simulink model "myexp8_3"  (R2022a)
settings: Solver=VariableStepAuto  StartTime=0.0  StopTime=10  RelTol=1e-3
undefined symbols (not defined in the file or in its folder): m, Q
libraries: commblkcod2 x2, commfilt2 x2, commdigbbndam3 x2, commchan3 x1, commrandsrc3 x1, commsink2 x1, dspsigops x1
settings Model: Creator=惠普  LastModifiedBy=惠普

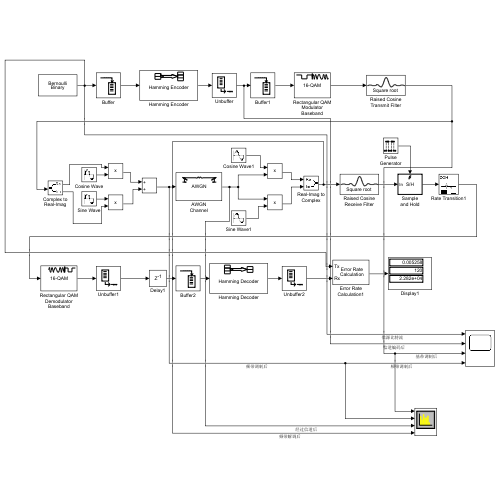
[thumbnail: Simulink's stored preview of the top-level diagram]
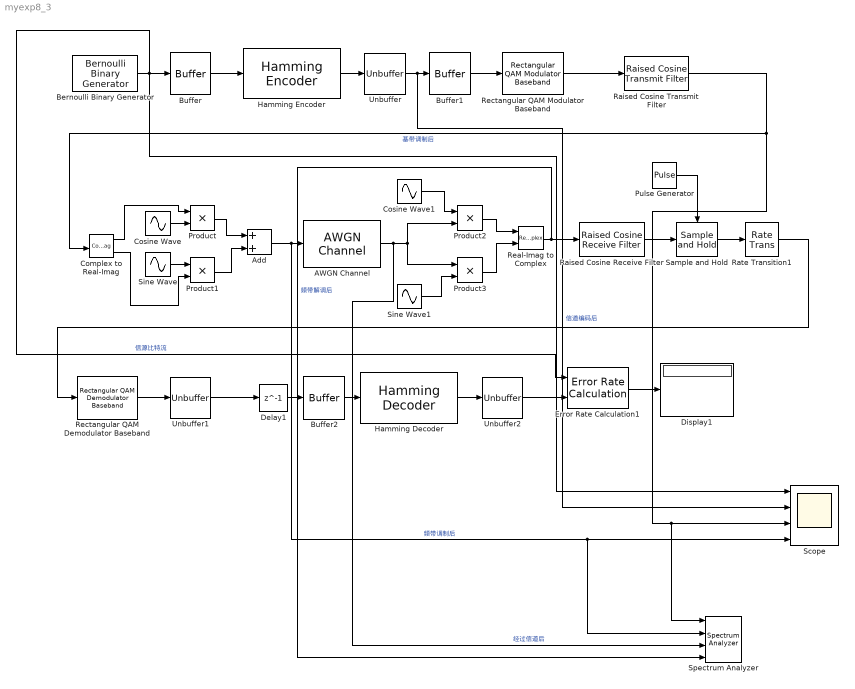
== system myexp8_3 ==
  AWGN Channel : commchan3/AWGN Channel  InputProcessing=Columns as channels (frame based)  seed=137  noiseMode="Signal to noise ratio  (Es/No)"  EbNodB=SNR  EsNodB=12  SNRdB=10  bitsPerSym=k  Ps=1  Tsym=1e-3  variance=1
  Add : Sum
  Bernoulli Binary Generator : commrandsrc3/Bernoulli Binary Generator  ProbabilityOfZero=0.5  SeedSource=Auto  Seed=0  SampleTime=1e-3*(2^m-1)/log2(Q)/(2^m-m-1)  SamplesPerFrame=1  OutputDataType=double  SimulateUsing=Interpreted execution
  Buffer : Buffer  N=2^m-m-1  OutputFrames=off
  Buffer1 : Buffer  N=log2(Q)  OutputFrames=off
  Buffer2 : Buffer  N=2^m-1  OutputFrames=off
  Complex to Real-Imag : ComplexToRealImag
  Cosine Wave : Sin  Amplitude=sqrt(2)  Frequency=2*pi*(10e3)  Phase=pi/2  SampleTime=1e-6
  Cosine Wave1 : Sin  Amplitude=sqrt(2)  Frequency=2*pi*(10e3)  Phase=pi/2  SampleTime=1e-6
  Delay1 : Delay  DelayLength=1  InitialCondition=0
  Display1 : Display
  Error Rate Calculation1 : commsink2/Error Rate Calculation  N=36  st_delay=0  cp_mode=Entire frame  subframe=[]  PMode=Port  WsName=ErrorVec  RsMode2=off  stop=off  numErr=100  maxBits=1e6
  Hamming Decoder : commblkcod2/Hamming Decoder  n=2^m-1  k=2^m-m-1
      settings: SourceProductBaseCode=CM
  Hamming Encoder : commblkcod2/Hamming Encoder  n=2^m-1  k=2^m-m-1
      settings: SourceProductBaseCode=CM
  Product{,1..3} (4 alike) : Product
  Pulse Generator : DiscretePulseGenerator  Period=1e3  PhaseDelay=10  SampleTime=1e-6
  Raised Cosine Receive Filter : commfilt2/Raised Cosine Receive Filter  filtType=Square root  R=0.5  filtSpan=10  N=1000  downFactor=1  downOffset=0  filterGain=1/sqrt(1000)  InputProcessing=Columns as channels (frame based)  RateOptions=Allow multirate processing  framing=Mute  checkCoeff=off  variableName=rcRxFilt1  currentFiltSpan=10  D=5  inputOffset=0  sampMode=Mute  saveAsFlag=0  rateMode=Downsampling  checkGain=Normalized  launchFVT=on  roundingMode=Floor  overflowMode=off  coeffDataTypeStr=Inherit: Same word length as input  coeffMin=[]  coeffMax=[]  coeffLastDataTypeStr=Inherit: Same word length as input  accumDataTypeStr=Inherit: Same as product output  accumLastDataTypeStr=Inherit: Same as product output  outputDataTypeStr=Inherit: Same as accumulator  outputMin=[]  outputMax=[]  outputLastDataTypeStr=Inherit: Same as accumulator
  Raised Cosine Transmit Filter : commfilt2/Raised Cosine Transmit Filter  filtType=Square root  R=0.5  filtSpan=10  N=1000  filterGain=sqrt(1000)  InputProcessing=Columns as channels (frame based)  RateOptions=Allow multirate processing  framing=Mute  checkCoeff=off  variableName=rcTxFilt1  checkGain=Normalized  sampMode=Mute  saveAsFlag=0  currentFiltSpan=10  D=(10)/2  launchFVT=on  roundingMode=Floor  overflowMode=off  coeffDataTypeStr=Inherit: Same word length as input  coeffMin=[]  coeffMax=[]  coeffLastDataTypeStr=Inherit: Same word length as input  outputDataTypeStr=Inherit: Same as accumulator  outputMin=[]  outputMax=[]  outputLastDataTypeStr=Inherit: Same as accumulator
  Rate Transition1 : RateTransition  OutPortSampleTime=1e-3
  Real-Imag to Complex : RealImagToComplex
  Rectangular QAM Demodulator Baseband : commdigbbndam3/Rectangular QAM Demodulator Baseband  M=Q  OutType=Bit  DecType=Hard decision  VarSource=Dialog  Variance=1  Dec=Gray  Mapping=[0:15]  PowType=Average Power  MinDist=2  AvgPow=1  PeakPow=1  Ph=0  outDtype1=Inherit via internal rule  outDtype2=Inherit via internal rule  derotateFactorWordLen=16  derotateFactorDataTypeStr=Inherit: Same word length as input  derotateFactorLastDataTypeStr=Inherit: Same word length as input  denormFactorWordLen=16  denormFactorDataTypeStr=Inherit: Same word length as input  denormFactorLastDataTypeStr=Inherit: Same word length as input  prodOutWordLen=32  prodOutOverflowMode=Wrap  prodOutRoundingMode=Floor  prodOutOvFlMode=off  prodOutOvFlModeLastStrValue=off  sumWordLen=32
  Rectangular QAM Modulator Baseband : commdigbbndam3/Rectangular QAM Modulator Baseband  M=Q  InType=Bit  Enc=Gray  Mapping=[0:15]  PowType=Average Power  MinDist=2  AvgPow=1  PeakPow=1  Ph=0  outDtype=double  outWordLen=16  outUDDataType=sfix(16)  outFracLenMode=Best precision  outFracLen=15  outDataTypeStr=double  outLastDataTypeStr=double
  Sample and Hold : dspsigops/Sample and Hold  trig=Rising edge  initCond=0  latchinput=off
  Scope : Scope  NumInputPorts=4
  Sine Wave : Sin  Amplitude=sqrt(2)  Frequency=2*pi*(10e3)  Phase=pi  SampleTime=1e-6
  Sine Wave1 : Sin  Amplitude=sqrt(2)  Frequency=2*pi*(10e3)  Phase=pi  SampleTime=1e-6
  Spectrum Analyzer : SpectrumAnalyzer  NumInputPorts=4
  Unbuffer : Unbuffer
  Unbuffer1 : Unbuffer
  Unbuffer2 : Unbuffer
  wires:
  Unbuffer2/1 -> Error Rate Calculation1/2
  Bernoulli Binary Generator/1 -> Scope/1, Error Rate Calculation1/1, Buffer/1  "信源比特流"
  Error Rate Calculation1/1 -> Display1/1
  Hamming Encoder/1 -> Unbuffer/1
  Buffer/1 -> Hamming Encoder/1
  Rectangular QAM Modulator Baseband/1 -> Raised Cosine Transmit Filter/1
  Complex to Real-Imag/1 -> Product/1
  Sine Wave/1 -> Product1/1
  Product1/1 -> Add/2
  Cosine Wave/1 -> Product/2
  Product/1 -> Add/1
  Complex to Real-Imag/2 -> Product1/2
  Add/1 -> Spectrum Analyzer/2, Scope/4, AWGN Channel/1  "频带调制后"
  AWGN Channel/1 -> Spectrum Analyzer/3, Product3/1, Product2/2  "经过信道后"
  Cosine Wave1/1 -> Product2/1
  Product3/1 -> Real-Imag to Complex/2
  Sine Wave1/1 -> Product3/2
  Product2/1 -> Real-Imag to Complex/1
  Pulse Generator/1 -> Sample and Hold/Trigger
  Raised Cosine Receive Filter/1 -> Sample and Hold/1
  Sample and Hold/1 -> Rate Transition1/1
  Rate Transition1/1 -> Rectangular QAM Demodulator Baseband/1
  Real-Imag to Complex/1 -> Spectrum Analyzer/4, Raised Cosine Receive Filter/1  "频带解调后"
  Rectangular QAM Demodulator Baseband/1 -> Unbuffer1/1
  Hamming Decoder/1 -> Unbuffer2/1
  Raised Cosine Transmit Filter/1 -> Spectrum Analyzer/1, Scope/3, Complex to Real-Imag/1  "基带调制后"
  Buffer2/1 -> Hamming Decoder/1
  Unbuffer/1 -> Scope/2, Buffer1/1  "信道编码后"
  Buffer1/1 -> Rectangular QAM Modulator Baseband/1
  Unbuffer1/1 -> Delay1/1
  Delay1/1 -> Buffer2/1
